simulink model "LKA_Lenkung_CarMaker_DSR_kombiniert"  (Simulink 7.9)
settings: Solver=ode23  StartTime=0.0  StopTime=tend  FixedStep=0.01  RelTol=1e-3
undefined symbols (not defined in the file or in its folder): contr, pin
libraries: library x6, simulink x6
settings Model: Creator=Georg  LastModifiedBy=Georg
settings DebuggingCC: FcnCallInpInsideContextMsg=Use local settings
settings GRTTargetCC: CombineOutputUpdateFcns=off  GRTInterface=on

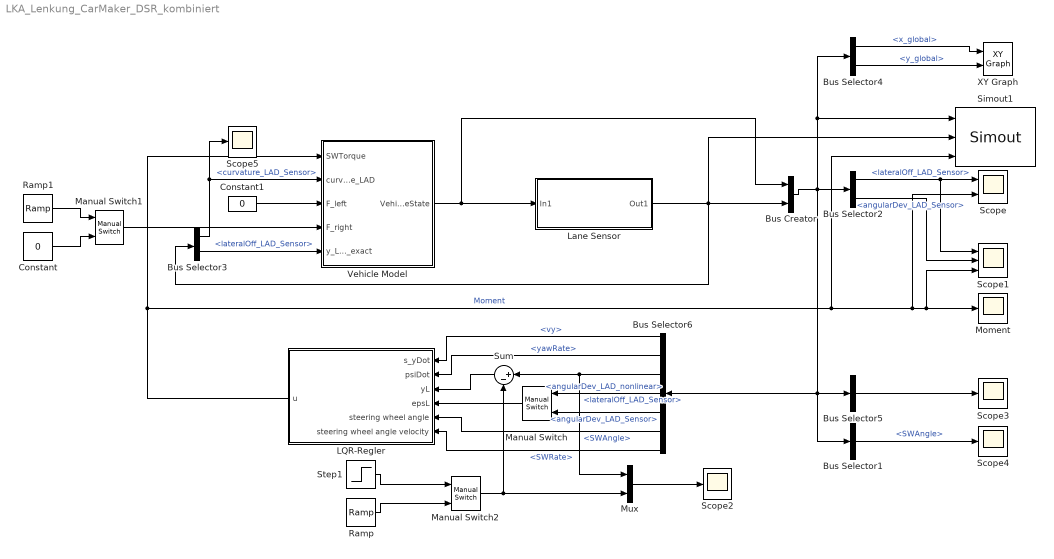
== system LKA_Lenkung_CarMaker_DSR_kombiniert ==
  Bus Creator : BusCreator  Inputs=2
  Bus Selector1 : BusSelector  OutputSignals=VehicleState.SWAngle
  Bus Selector2 : BusSelector  OutputSignals=LaneSensor.lateralOff_LAD_Sensor,LaneSensor.angularDev_LAD_Sensor
  Bus Selector3 : BusSelector  OutputSignals=curvature_LAD_Sensor,lateralOff_LAD_Sensor
  Bus Selector4 : BusSelector  OutputSignals=VehicleState.x_global,VehicleState.y_global
  Bus Selector5 : BusSelector  OutputSignals=VehicleState.angularDev_LAD_nonlinear,LaneSensor.angularDev_LAD_Sensor  OutputAsBus=on
  Bus Selector6 : BusSelector  OutputSignals=VehicleState.vy,VehicleState.yawRate,LaneSensor.lateralOff_LAD_Sensor,VehicleState.angularDev_LAD_nonlinear,LaneSensor.angularDev_LAD_Sensor,VehicleState.SWAngle,VehicleState.SWRate
  Constant : Constant  Value=0
  Constant1 : Constant  Value=0
  LQR-Regler : Subsystem
  Lane Sensor : Subsystem
  Manual Switch : simulink/Signal Routing/Manual Switch  sw=1  action=0  varsize=off
  Manual Switch1 : simulink/Signal Routing/Manual Switch  sw=0  action=0  varsize=off
  Manual Switch2 : simulink/Signal Routing/Manual Switch  sw=1  action=0  varsize=off
  Moment : Scope
      settings: TimeRange=33.61  YMin=-0.001  YMax=0.011  SaveName=ScopeData2
  Mux : Mux  Inputs=2
  Ramp : simulink/Sources/Ramp  slope=1  start=10  X0=0
  Ramp1 : simulink/Sources/Ramp  slope=1  start=10  X0=0
  Scope : Scope  NumInputPorts=2
      settings: TimeRange=45  YMin=-0.0002~0  YMax=0.0012~0.0002
  Scope1 : Scope  NumInputPorts=3
      settings: TimeRange=20  YMin=-5.5e-008~0.01711~-1.666e-008  YMax=5e-009~0.017145~-1.6565e-008
  Scope{2..5} (4 alike) : Scope
      Scope2 settings: YMin=-5e-005  YMax=0.0011  SaveName=ScopeData5
      Scope3 settings: ShowLegends=on  YMin=-1.75  YMax=0.25  SaveName=ScopeData3
      Scope4 settings: YMin=0.00625  YMax=0.0095  SaveName=ScopeData4
      Scope5 settings: YMin=0.00475  YMax=0.00525  SaveName=ScopeData6
  Simout1 : library/Misc/Simout
  Step1 : Step  Time=10  After=0  SampleTime=0
  Sum : Sum  Inputs=|+-
  Vehicle Model : Subsystem
  XY Graph : simulink/Sinks/XY Graph  xmin=-100  xmax=700  ymin=-1  ymax=600  st=-1
  wires:
  Bus Selector4/1 -> XY Graph/1  "<x_global>"
  Bus Selector4/2 -> XY Graph/2  "<y_global>"
  LQR-Regler/1(u) -> Vehicle Model/1(SWTorque), Scope/2, Scope1/3, Moment/1, Simout1/3  "Moment"
  Bus Selector2/1 -> Scope/1, Scope1/1  "<lateralOff_LAD_Sensor>"
  Bus Selector2/2 -> Scope1/2  "<angularDev_LAD_Sensor>"
  Vehicle Model/1(VehicleState) -> Bus Creator/1, Lane Sensor/1(In1)
  Lane Sensor/1(Out1) -> Bus Creator/2, Bus Selector3/1, Simout1/2
  Bus Creator/1 -> Bus Selector2/1, Bus Selector5/1, Bus Selector6/1, Bus Selector1/1, Bus Selector4/1, Simout1/1
  Bus Selector5/1 -> Scope3/1
  Bus Selector1/1 -> Scope4/1  "<SWAngle>"
  Ramp1/1 -> Manual Switch1/1
  Constant/1 -> Manual Switch1/2
  Bus Selector6/4 -> Manual Switch/1  "<angularDev_LAD_nonlinear>"
  Bus Selector6/5 -> Manual Switch/2  "<angularDev_LAD_Sensor>"
  Manual Switch1/1 -> Vehicle Model/4(F_right)
  Bus Selector3/1 -> Scope5/1, Vehicle Model/2(curvature_LAD)  "<curvature_LAD_Sensor>"
  Bus Selector6/1 -> LQR-Regler/1(s_yDot)  "<vy>"
  Bus Selector6/2 -> LQR-Regler/2(psiDot)  "<yawRate>"
  Bus Selector6/6 -> LQR-Regler/5(steering wheel angle)  "<SWAngle>"
  Bus Selector6/7 -> LQR-Regler/6(steering wheel angle velocity)  "<SWRate>"
  Manual Switch/1 -> LQR-Regler/4(epsL)
  Bus Selector6/3 -> Sum/1, Mux/1  "<lateralOff_LAD_Sensor>"
  Sum/1 -> LQR-Regler/3(yL)
  Manual Switch2/1 -> Sum/2, Mux/2
  Mux/1 -> Scope2/1
  Constant1/1 -> Vehicle Model/3(F_left)
  Step1/1 -> Manual Switch2/1
  Ramp/1 -> Manual Switch2/2
  Bus Selector3/2 -> Vehicle Model/5(y_LAD_exact)  "<lateralOff_LAD_Sensor>"

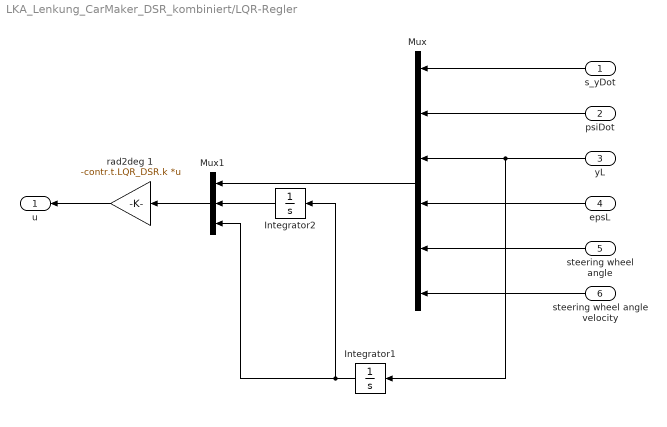
== system LKA_Lenkung_CarMaker_DSR_kombiniert/LQR-Regler ==
  s_yDot : Inport
  psiDot : Inport  Port=2
  yL : Inport  Port=3
  epsL : Inport  Port=4
  steering wheel angle : Inport  Port=5
  steering wheel angle velocity : Inport  Port=6
  Integrator1 : Integrator
  Integrator2 : Integrator
  Mux : Mux  Inputs=6
  Mux1 : Mux  Inputs=3
  rad2deg 1 : Gain  Gain=-contr.t.LQR_DSR.k  Multiplication=Matrix(K*u) (u vector)
  u : Outport
  wires:
  Mux/1 -> Mux1/1
  Mux1/1 -> rad2deg 1/1
  yL/1 -> Mux/3, Integrator1/1
  s_yDot/1 -> Mux/1
  psiDot/1 -> Mux/2
  rad2deg 1/1 -> u/1
  epsL/1 -> Mux/4
  steering wheel angle/1 -> Mux/5
  steering wheel angle velocity/1 -> Mux/6
  Integrator2/1 -> Mux1/2
  Integrator1/1 -> Integrator2/1, Mux1/3

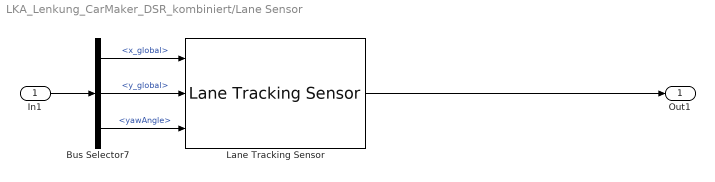
== system LKA_Lenkung_CarMaker_DSR_kombiniert/Lane Sensor ==
  In1 : Inport
  Bus Selector7 : BusSelector  OutputSignals=x_global,y_global,yawAngle
  Lane Tracking Sensor : library/Lane Tracking/Lane Tracking Sensor
  Out1 : Outport
  wires:
  Bus Selector7/1 -> Lane Tracking Sensor/1  "<x_global>"
  Bus Selector7/2 -> Lane Tracking Sensor/2  "<y_global>"
  Bus Selector7/3 -> Lane Tracking Sensor/3  "<yawAngle>"
  In1/1 -> Bus Selector7/1
  Lane Tracking Sensor/1 -> Out1/1

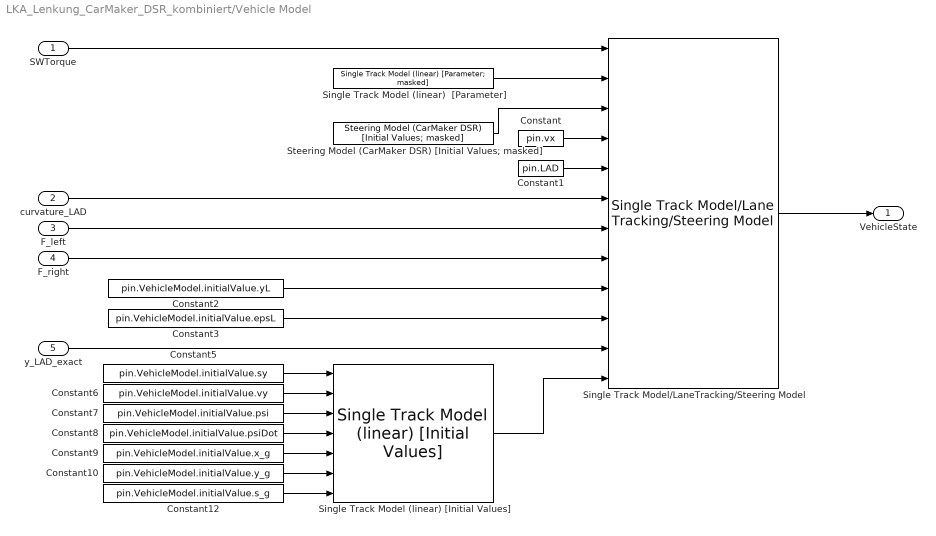
== system LKA_Lenkung_CarMaker_DSR_kombiniert/Vehicle Model ==
  SWTorque : Inport
  curvature_LAD : Inport  Port=2
  F_left : Inport  Port=3
  F_right : Inport  Port=4
  y_LAD_exact : Inport  Port=5
  Constant : Constant  Value=pin.vx
  Constant1 : Constant  Value=pin.LAD
  Constant10 : Constant  Value=pin.VehicleModel.initialValue.y_g
  Constant12 : Constant  Value=pin.VehicleModel.initialValue.s_g
  Constant2 : Constant  Value=pin.VehicleModel.initialValue.yL
  Constant3 : Constant  Value=pin.VehicleModel.initialValue.epsL
  Constant5 : Constant  Value=pin.VehicleModel.initialValue.sy
  Constant6 : Constant  Value=pin.VehicleModel.initialValue.vy
  Constant7 : Constant  Value=pin.VehicleModel.initialValue.psi
  Constant8 : Constant  Value=pin.VehicleModel.initialValue.psiDot
  Constant9 : Constant  Value=pin.VehicleModel.initialValue.x_g
  Single Track Model (linear) [Initial Values] : library/Vehicle Models ext./Single Track Model (linear) [Initial Values]
  Single Track Model (linear)  [Parameter] : library/Vehicle Models ext./Single Track Model (linear) [Parameter; masked]  cs_front=pin.VehicleModel.parameter.csv  cs_rear=pin.VehicleModel.parameter.csh  l_front=pin.VehicleModel.parameter.lv  l_rear=pin.VehicleModel.parameter.lh  m=pin.VehicleModel.parameter.m  Izz=pin.VehicleModel.parameter.Iz
  Single Track Model/LaneTracking/Steering Model : library/Vehicle Models ext./Single Track Model//Lane Tracking//Steering Model
  Steering Model (CarMaker DSR) [Initial Values; masked] : library/Vehicle Models ext./Steering Model (CarMaker DSR) [Initial Values; masked]  d_rot=pin.SteeringModel.parameter.drot  d_rack=pin.SteeringModel.parameter.drack  i_HR=pin.SteeringModel.parameter.iHR  I_rot=pin.SteeringModel.parameter.J  m_left=pin.SteeringModel.parameter.mL  m_right=pin.SteeringModel.parameter.mR  m_rack=pin.SteeringModel.parameter.mr  V=pin.SteeringModel.parameter.V  alpha=pin.SteeringModel.parameter.alph
  VehicleState : Outport
  wires:
  curvature_LAD/1 -> Single Track Model/LaneTracking/Steering Model/6
  Steering Model (CarMaker DSR) [Initial Values; masked]/1 -> Single Track Model/LaneTracking/Steering Model/3
  Constant/1 -> Single Track Model/LaneTracking/Steering Model/4
  Constant1/1 -> Single Track Model/LaneTracking/Steering Model/5
  Single Track Model/LaneTracking/Steering Model/1 -> VehicleState/1
  F_left/1 -> Single Track Model/LaneTracking/Steering Model/7
  F_right/1 -> Single Track Model/LaneTracking/Steering Model/8
  Constant2/1 -> Single Track Model/LaneTracking/Steering Model/9
  Constant3/1 -> Single Track Model/LaneTracking/Steering Model/10
  y_LAD_exact/1 -> Single Track Model/LaneTracking/Steering Model/11
  SWTorque/1 -> Single Track Model/LaneTracking/Steering Model/1
  Single Track Model (linear)  [Parameter]/1 -> Single Track Model/LaneTracking/Steering Model/2
  Constant5/1 -> Single Track Model (linear) [Initial Values]/1
  Constant6/1 -> Single Track Model (linear) [Initial Values]/2
  Constant7/1 -> Single Track Model (linear) [Initial Values]/3
  Constant8/1 -> Single Track Model (linear) [Initial Values]/4
  Constant9/1 -> Single Track Model (linear) [Initial Values]/5
  Constant10/1 -> Single Track Model (linear) [Initial Values]/6
  Constant12/1 -> Single Track Model (linear) [Initial Values]/7
  Single Track Model (linear) [Initial Values]/1 -> Single Track Model/LaneTracking/Steering Model/12
